simulink model "kvadrokopter"  (R2015b)
settings: Solver=VariableStepAuto  StartTime=0.0  StopTime=240  FixedStep=0.001  MaxStep=0.1  RelTol=1e-3
libraries: simulink x6
settings Model: Creator=DNikolaev  LastModifiedBy=DNikolaev

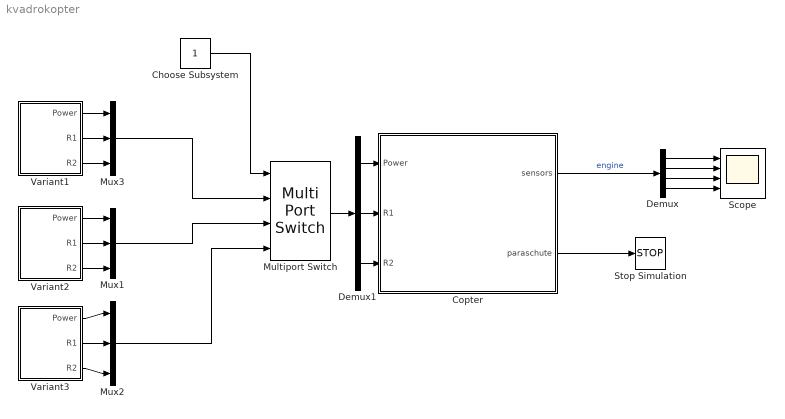
== system kvadrokopter ==
  Choose Subsystem : Constant
  Copter : Stateflow chart  TreatAsAtomicUnit=on
  Demux : Demux
  Demux1 : Demux  Outputs=3
  Multiport Switch : MultiPortSwitch
  Mux1 : Mux  Inputs=3
  Mux2 : Mux  Inputs=3
  Mux3 : Mux  Inputs=3
  Scope : Scope  NumInputPorts=4
  Stop Simulation : Stop
  Variant1 : Subsystem
  Variant2 : Subsystem
  Variant3 : Subsystem
  wires:
  Copter/2(paraschute) -> Stop Simulation/1
  Copter/1(sensors) -> Demux/1  "engine"
  Demux/2 -> Scope/2
  Demux/3 -> Scope/3
  Demux/1 -> Scope/1
  Demux/4 -> Scope/4
  Multiport Switch/1 -> Demux1/1
  Demux1/2 -> Copter/2(R1)
  Demux1/1 -> Copter/1(Power)
  Demux1/3 -> Copter/3(R2)
  Variant3/1("Power ") -> Mux2/1
  Variant3/2(R1) -> Mux2/2
  Variant3/3(R2) -> Mux2/3
  Variant2/1("Power ") -> Mux1/1
  Variant2/2(R1) -> Mux1/2
  Variant2/3(R2) -> Mux1/3
  Variant1/3(R2) -> Mux3/3
  Variant1/2(R1) -> Mux3/2
  Variant1/1("Power ") -> Mux3/1
  Mux3/1 -> Multiport Switch/2
  Mux1/1 -> Multiport Switch/3
  Mux2/1 -> Multiport Switch/4
  Choose Subsystem/1 -> Multiport Switch/1

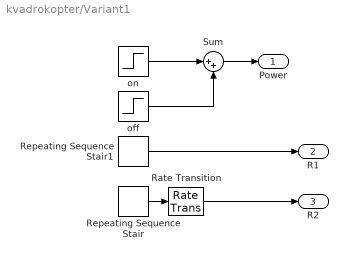
== system kvadrokopter/Variant1 ==
  Rate Transition : RateTransition
  Repeating Sequence Stair : simulink/Sources/Repeating Sequence Stair  OutValues=[0 0 0 1 2 3 4 5 6 7 8]  tsamp=10  OutMin=[]  OutMax=[]  OutDataTypeStr=double  OutputDataTypeScalingMode=double  OutDataType=fixdt(0,8)  ConRadixGroup=Best Precision: Vector-wise  OutScaling=2^-12
  Repeating Sequence Stair1 : simulink/Sources/Repeating Sequence Stair  OutValues=[2 3 2 2 2 2 2 2 2 2 2 2 2 2 1 1 1 1 1 1 1 1 1 1 1 1 1 1 ]  tsamp=10  OutMin=[]  OutMax=[]  OutDataTypeStr=double  OutputDataTypeScalingMode=double  OutDataType=fixdt(0,8)  ConRadixGroup=Best Precision: Vector-wise  OutScaling=2^-12
  Sum : Sum  Inputs=|++
  off : Step  Time=200  After=-1  SampleTime=0
  on : Step  Time=10  SampleTime=0
  "Power " : Outport
  R1 : Outport  Port=2
  R2 : Outport  Port=3
  wires:
  Repeating Sequence Stair1/1 -> R1/1
  Repeating Sequence Stair/1 -> Rate Transition/1
  on/1 -> Sum/1
  Rate Transition/1 -> R2/1
  off/1 -> Sum/2
  Sum/1 -> "Power "/1

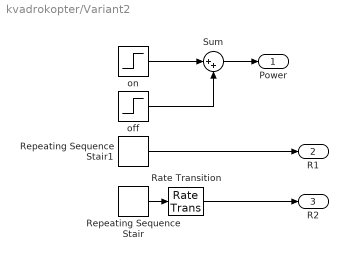
== system kvadrokopter/Variant2 ==
  Rate Transition : RateTransition
  Repeating Sequence Stair : simulink/Sources/Repeating Sequence Stair  OutValues=[0 0 0 1 0]  tsamp=10  OutMin=[]  OutMax=[]  OutDataTypeStr=double  OutputDataTypeScalingMode=double  OutDataType=fixdt(0,8)  ConRadixGroup=Best Precision: Vector-wise  OutScaling=2^-12
  Repeating Sequence Stair1 : simulink/Sources/Repeating Sequence Stair  OutValues=[2 3 2 2 2 2 2 2 2 2 2 2 2 2 2 2 2 2 2 2 2 2 ]  tsamp=10  OutMin=[]  OutMax=[]  OutDataTypeStr=double  OutputDataTypeScalingMode=double  OutDataType=fixdt(0,8)  ConRadixGroup=Best Precision: Vector-wise  OutScaling=2^-12
  Sum : Sum  Inputs=|++
  off : Step  Time=50  After=-1  SampleTime=0
  on : Step  Time=10  SampleTime=0
  "Power " : Outport
  R1 : Outport  Port=2
  R2 : Outport  Port=3
  wires:
  Sum/1 -> "Power "/1
  off/1 -> Sum/2
  Rate Transition/1 -> R2/1
  on/1 -> Sum/1
  Repeating Sequence Stair/1 -> Rate Transition/1
  Repeating Sequence Stair1/1 -> R1/1

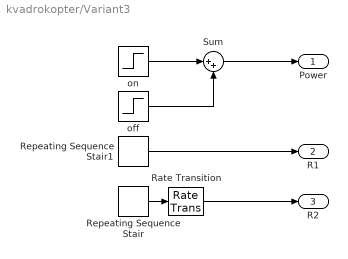
== system kvadrokopter/Variant3 ==
  Rate Transition : RateTransition
  Repeating Sequence Stair : simulink/Sources/Repeating Sequence Stair  OutValues=[0 0 0 1 2 3 4 5 6 7 8]  tsamp=10  OutMin=[]  OutMax=[]  OutDataTypeStr=double  OutputDataTypeScalingMode=double  OutDataType=fixdt(0,8)  ConRadixGroup=Best Precision: Vector-wise  OutScaling=2^-12
  Repeating Sequence Stair1 : simulink/Sources/Repeating Sequence Stair  OutValues=[2 2 2 2 3 2 2 1 3 2 2 2 2 2 2 2 ]  tsamp=10  OutMin=[]  OutMax=[]  OutDataTypeStr=double  OutputDataTypeScalingMode=double  OutDataType=fixdt(0,8)  ConRadixGroup=Best Precision: Vector-wise  OutScaling=2^-12
  Sum : Sum  Inputs=|++
  off : Step  Time=160  After=-1  SampleTime=0
  on : Step  Time=10  SampleTime=0
  "Power " : Outport
  R1 : Outport  Port=2
  R2 : Outport  Port=3
  wires:
  Sum/1 -> "Power "/1
  off/1 -> Sum/2
  Rate Transition/1 -> R2/1
  on/1 -> Sum/1
  Repeating Sequence Stair/1 -> Rate Transition/1
  Repeating Sequence Stair1/1 -> R1/1

== stateflow chart kvadrokopter/Copter ==
  state Avariynaya_posadka
    entry:
    paraschute=1;
    sensors=[0 0 0 0];
    engines=[0 0 0 0];
  state PowerOff
    entry:
    sensors=[0 0 0 0];
    engines=[0 0 0 0];
    paraschute=0;
  state PowerOn
    entry: engines=[2 2 2 2];
    fly=0;
    state Rychagi [parallel]
      settings: executionOrder=2
      state Zavisanie
        entry: engines=[2 2 2 2];
      state Posadka
        entry: engines=[1 1 1 1];
        fly=0;
      state Vzlet
        entry: engines=[3 3 3 3];
        fly=1;
      state Vpered
        entry: engines=[1 1 3 3];
      state Nazad
        entry: engines=[3 3 1 1];
      state Vlevo
        entry: engines=[1 3 3 1];
      state Vpravo
        entry: engines=[3 1 1 3];
      state Vverh
        entry: engines=[3 3 3 3];
      state Vniz
        entry: engines=[1 1 1 1];
      state Pochasovoy
        entry: engines=[1 3 1 3];
      state Protivchasovoy1
        entry: engines=[3 1 3 1];
      (junction 247) -> Posadka [order 2] : [R1==1]
      Posadka -> (junction 322) [order 2] : [R1~=1]
      (junction 317) -> (junction 322) [order 2] : [R2==0]
      (junction 322) -> Zavisanie
      (default) -> Zavisanie
      Vzlet -> (junction 322) [order 2] : [R1~=3]
      (junction 247) -> Vzlet [order 1] : [R1==3]
      Zavisanie -> (junction 247) [order 2]
      (junction 245) -> (junction 247)
      Zavisanie -> (junction 170) [order 1] : [fly==1]
      (junction 179) -> (junction 317)
      (junction 317) -> (junction 170) [order 1]
      (junction 170) -> Posadka [order 1] : [R1==1]
      (junction 170) -> Vzlet [order 2] : [R1==3]
      Vzlet -> (junction 245) [order 1]
      (junction 170) -> (junction 174) [order 3]
      (junction 243) -> (junction 245)
      (junction 174) -> Vpered [order 1] : [R2==1]
      Vpered -> (junction 179) [order 1] : [R2~=1]
      (junction 174) -> (junction 203) [order 2]
      (junction 182) -> (junction 179)
      Vpered -> (junction 243) [order 2]
      (junction 241) -> (junction 243)
      (junction 203) -> Nazad [order 1] : [R2==2]
      Nazad -> (junction 182) [order 1] : [R2~=2]
      (junction 203) -> (junction 205) [order 2]
      (junction 184) -> (junction 182)
      Nazad -> (junction 241) [order 2]
      (junction 239) -> (junction 241)
      Vlevo -> (junction 184) [order 1] : [R2~=3]
      (junction 205) -> Vlevo [order 1] : [R2==3]
      (junction 186) -> (junction 184)
      (junction 205) -> (junction 207) [order 2]
      Vlevo -> (junction 239) [order 2]
      (junction 237) -> (junction 239)
      Vpravo -> (junction 186) [order 1] : [R2~=4]
      (junction 207) -> Vpravo [order 1] : [R2==4]
      (junction 188) -> (junction 186)
      (junction 207) -> (junction 209) [order 2]
      Vpravo -> (junction 237) [order 2]
      (junction 235) -> (junction 237)
      (junction 209) -> Vverh [order 1] : [R2==5]
      Vverh -> (junction 188) [order 1] : [R2~=5]
      (junction 209) -> (junction 211) [order 2]
      (junction 190) -> (junction 188)
      Vverh -> (junction 235) [order 2]
      (junction 233) -> (junction 235)
      Vniz -> (junction 190) [order 1] : [R2~=6]
      (junction 211) -> Vniz [order 1] : [R2==6]
      (junction 192) -> (junction 190)
      (junction 211) -> (junction 213) [order 2]
      Vniz -> (junction 233) [order 2]
      (junction 231) -> (junction 233)
      Pochasovoy -> (junction 192) [order 1] : [R2~=7]
      (junction 213) -> Pochasovoy [order 1] : [R2==7]
      (junction 194) -> (junction 192)
      (junction 213) -> (junction 215) [order 2]
      Pochasovoy -> (junction 231) [order 2]
      (junction 229) -> (junction 231)
      (junction 215) -> Protivchasovoy1 : [R2==8]
      Protivchasovoy1 -> (junction 194) [order 1] : [R2~=8]
      Protivchasovoy1 -> (junction 229) [order 2]
    state Engine1 [parallel]
      settings: executionOrder=1
      state Low
        en: sensors(1)=1;
      state Medium
        en: sensors(1)=2;
      state High
        en: sensors(1)=3;
      (junction 117) -> PowerOn.Engine1.Low [order 1] : [engines(1)==1]
      PowerOn.Engine1.Low -> (junction 149) : [engines(1)~=1]
      PowerOn.Engine1.Medium -> (junction 149) : [engines(1)~=2]
      (default) -> (junction 117)
      (junction 117) -> PowerOn.Engine1.Medium [order 2] : [engines(1)==2]
      (junction 117) -> PowerOn.Engine1.High [order 3] : [engines(1)==3]
      PowerOn.Engine1.High -> (junction 149) : [engines(1)~=3]
      (junction 149) -> (junction 117)
    state Engine2 [parallel]
      settings: executionOrder=3
      state Low
        en: sensors(2)=1;
      state Medium
        en: sensors(2)=2;
      state High
        en: sensors(2)=3;
      (junction 279) -> PowerOn.Engine2.Low [order 1] : [engines(2)==1]
      PowerOn.Engine2.Low -> (junction 276) : [engines(2)~=1]
      PowerOn.Engine2.Medium -> (junction 276) : [engines(2)~=2]
      (default) -> (junction 279)
      (junction 279) -> PowerOn.Engine2.Medium [order 2] : [engines(2)==2]
      (junction 279) -> PowerOn.Engine2.High [order 3] : [engines(2)==3]
      PowerOn.Engine2.High -> (junction 276) : [engines(2)~=3]
      (junction 276) -> (junction 279)
    state Engine3 [parallel]
      settings: executionOrder=4
      state Low
        en: sensors(3)=1;
      state Medium
        en: sensors(3)=2;
      state High
        en: sensors(3)=3;
      (junction 293) -> PowerOn.Engine3.Low [order 1] : [engines(3)==1]
      PowerOn.Engine3.Low -> (junction 290) : [engines(3)~=1]
      PowerOn.Engine3.Medium -> (junction 290) : [engines(3)~=2]
      (default) -> (junction 293)
      (junction 293) -> PowerOn.Engine3.Medium [order 2] : [engines(3)==2]
      (junction 293) -> PowerOn.Engine3.High [order 3] : [engines(3)==3]
      PowerOn.Engine3.High -> (junction 290) : [engines(3)~=3]
      (junction 290) -> (junction 293)
    state Engine4 [parallel]
      settings: executionOrder=5
      state Low
        en: sensors(4)=1;
      state Medium
        en: sensors(4)=2;
      state High
        en: sensors(4)=3;
      (junction 307) -> PowerOn.Engine4.Low [order 1] : [engines(4)==1]
      PowerOn.Engine4.Low -> (junction 304) : [engines(4)~=1]
      PowerOn.Engine4.Medium -> (junction 304) : [engines(4)~=2]
      (default) -> (junction 307)
      (junction 307) -> PowerOn.Engine4.Medium [order 2] : [engines(4)==2]
      (junction 307) -> PowerOn.Engine4.High [order 3] : [engines(4)==3]
      PowerOn.Engine4.High -> (junction 304) : [engines(4)~=3]
      (junction 304) -> (junction 307)
  (default) -> PowerOff
  PowerOn -> Avariynaya_posadka : [Power==0 && fly==1]
  Posadka -> PowerOff [order 1] : [Power==0]
  PowerOff -> PowerOn : [Power==1]
  data: sensors output; engines local; paraschute output; Power input; R1 input; R2 input; fly local
